simulink model "pid_pith"  (Simulink 5.0)
settings: Solver=ode5  StartTime=0.0  StopTime=75  FixedStep=.01  RelTol=1e-3
values from neighbouring files (symbols this model uses):
  control_p = [-1 -0.975 -0.95 -0.925 -0.9 -0.875 -0.85 -0.825 -0.8 -0.775 -0.75 -0.725 ... (81 elements, 1x81)]    [tras_char.mat]
  force_p = [-0.71417078206 -0.698541481137 -0.676359428972 -0.657306593399 -0.636149510201 -0.615949677515 -0.602138570677 -0.585879142379 -0.565408182885 -0.543655801355 -0.527755120628 -0.502405059235 ... (81 elements, 1x81)]    [tras_char.mat]
  rpm_p = [-3678.29210985 -3557.9090356 -3500.75969748 -3468.48920637 -3408.40308809 -3364.59631401 -3305.24812764 -3268.16062475 -3204.9654373 -3137.29807834 -3101.82489983 -3044.64042209 ... (81 elements, 1x81)]    [tras_char.mat]
undefined symbols (not defined in the file or in its folder): a, b, c
settings Model: LastModifiedBy=Administrator

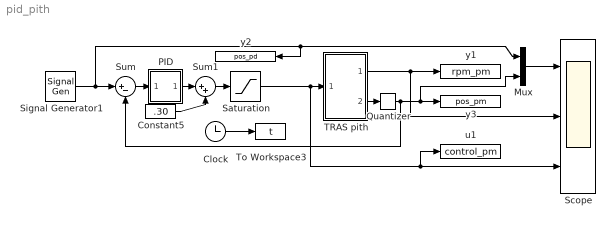
== system pid_pith ==
  Clock : Clock
  Constant5 : Constant  Value=.30
  Mux : Mux  Inputs=2
  "PID " : Subsystem  AncestorBlock=|  mask(PID(2) Controller){P=a, I=b, D=c, N=100, S=1.43}
      | simulink_extras/Additional
      | Linear/PID Controller
      | (with Approximate
      | Derivative)
      mask prompts: P "Proportional:"; I "Integral:"; D "Derivative:"; N "Derivative divisor(N):"; S "Integral sat (0-1)"
      mask help:
      | Enter Proportional(P), Integral(I), and Derivative(D) and divisor (N) terms.
      | P+I/s+Ds/(1/Ns+1)
      mask Help: This block implements a PID controller where parameters are entered for the Proportional, Integral and Derivative and divisor terms. Unmask this block to see how it works. The derivative term is implemented using an s/(s/N +1)  transfer function block. Making N large can create a "stiff" system.
      mask Display: disp('PID')
  Quantizer : Quantizer  QuantizationInterval=(2*pi)/4096
  Saturation : Saturate  UpperLimit=1  LowerLimit=.2
  Scope : Scope  NumInputPorts=3
      settings: YMin=-1.5~0~0  YMax=1~3000~1  MaxDataPoints=50000
  Signal Generator1 : SignalGenerator  WaveForm=square  Amplitude=.10  Frequency=.02
  Sum : Sum  Inputs=|+-  SaturateOnIntegerOverflow=on
  Sum1 : Sum  Inputs=|++  SaturateOnIntegerOverflow=on  InputSameDT=on
  TRAS pith : Subsystem
  To Workspace3 : ToWorkspace  VariableName=t  SampleTime=-1  SaveFormat=Array
  u1 : ToWorkspace  VariableName=control_pm  SampleTime=-1  SaveFormat=Array
  y1 : ToWorkspace  VariableName=rpm_pm  SampleTime=-1  SaveFormat=Array
  y2 : ToWorkspace  VariableName=pos_pd  SampleTime=-1  SaveFormat=Array
  y3 : ToWorkspace  VariableName=pos_pm  SampleTime=-1  SaveFormat=Array
  wires:
  TRAS pith/1(rpm_p) -> y1/1, Scope/2
  TRAS pith/2(pos_pm) -> Quantizer/1
  Clock/1 -> To Workspace3/1
  Signal Generator1/1 -> Sum/1, Mux/1, y2/1
  Sum/1 -> "PID "/1(In_1)
  Mux/1 -> Scope/1
  Saturation/1 -> TRAS pith/1(ctrl_p), Scope/3, u1/1
  "PID "/1(Out_1) -> Sum1/1
  Sum1/1 -> Saturation/1
  Constant5/1 -> Sum1/2
  Quantizer/1 -> y3/1, Mux/2, Sum/2

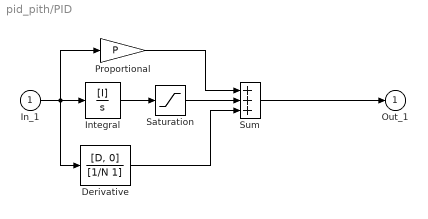
== system pid_pith/PID  ==
  In_1 : Inport
  Derivative : TransferFcn  Numerator=[D, 0]  Denominator=[1/N 1]
  Integral : TransferFcn  Numerator=[I]  Denominator=[1 0]
  Proportional : Gain  Gain=P  SaturateOnIntegerOverflow=on
  Saturation : Saturate  UpperLimit=S  LowerLimit=-S
  Sum : Sum  Inputs=+++  SaturateOnIntegerOverflow=on  InputSameDT=on
  Out_1 : Outport  InitialOutput=0
  wires:
  Sum/1 -> Out_1/1
  In_1/1 -> Derivative/1, Integral/1, Proportional/1
  Derivative/1 -> Sum/3
  Integral/1 -> Saturation/1
  Proportional/1 -> Sum/1
  Saturation/1 -> Sum/2

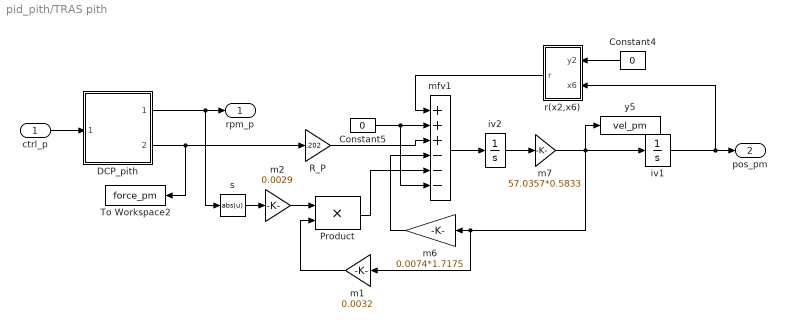
== system pid_pith/TRAS pith ==
  ctrl_p : Inport
  Constant4 : Constant  Orientation=left  Value=0
  Constant5 : Constant  Value=0
  DCP_pith : Subsystem
  Product : Product  SaturateOnIntegerOverflow=on
  R_P : Gain  Gain=.202
  To Workspace2 : ToWorkspace  VariableName=force_pm  SampleTime=-1  SaveFormat=Array
  iv1 : Integrator  InitialCondition=-.5319*0  UpperSaturationLimit=pi  LowerSaturationLimit=-pi
  iv2 : Integrator  InitialCondition=-.1  LimitOutput=on  UpperSaturationLimit=pi  LowerSaturationLimit=-pi
  m1 : Gain  Orientation=left  Gain=0.0032  SaturateOnIntegerOverflow=on
  m2 : Gain  Gain=0.0029  SaturateOnIntegerOverflow=on
  m6 : Gain  Orientation=left  Gain=0.0074*1.7175
  m7 : Gain  Gain=57.0357*0.5833  SaturateOnIntegerOverflow=on
  mfv1 : Sum  Inputs=+++---  SaturateOnIntegerOverflow=on  InputSameDT=on
  r(x2,x6) : Subsystem  Orientation=left
  s : Fcn  Expr=abs(u)
  y5 : ToWorkspace  VariableName=vel_pm  SampleTime=-1  SaveFormat=Array
  rpm_p : Outport
  pos_pm : Outport  Port=2
  wires:
  ctrl_p/1 -> DCP_pith/1(CTR_P)
  mfv1/1 -> iv2/1
  m2/1 -> Product/1
  m1/1 -> Product/2
  iv1/1 -> pos_pm/1, r(x2,x6)/2(x6)
  Constant5/1 -> mfv1/6, mfv1/2
  Constant4/1 -> r(x2,x6)/1(y2)
  R_P/1 -> mfv1/3
  r(x2,x6)/1(r) -> mfv1/1
  Product/1 -> mfv1/5
  s/1 -> m2/1
  DCP_pith/1(RPM_P) -> rpm_p/1, s/1
  m7/1 -> iv1/1, m1/1, m6/1, y5/1
  iv2/1 -> m7/1
  m6/1 -> mfv1/4
  DCP_pith/2(FORCE_P) -> R_P/1, To Workspace2/1

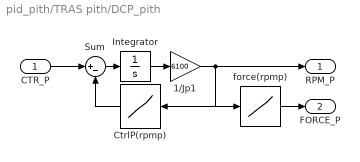
== system pid_pith/TRAS pith/DCP_pith ==
  CTR_P : Inport
  1/Jp1 : Gain  Gain=6100  ShowAdditionalParam=on
  CtrlP(rpmp) : Lookup  Orientation=left  InputValues=rpm_p  OutputValues=control_p  SaturateOnIntegerOverflow=on
  Integrator : Integrator
  Sum : Sum  Inputs=|+-  SaturateOnIntegerOverflow=on  InputSameDT=on
  force(rpmp) : Lookup  InputValues=rpm_p  OutputValues=force_p  SaturateOnIntegerOverflow=on
  RPM_P : Outport
  FORCE_P : Outport  Port=2
  wires:
  force(rpmp)/1 -> FORCE_P/1
  CTR_P/1 -> Sum/1
  1/Jp1/1 -> RPM_P/1, force(rpmp)/1, CtrlP(rpmp)/1
  CtrlP(rpmp)/1 -> Sum/2
  Integrator/1 -> 1/Jp1/1
  Sum/1 -> Integrator/1

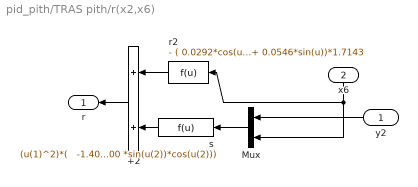
== system pid_pith/TRAS pith/r(x2,x6) ==
  y2 : Inport  Orientation=left
  x6 : Inport  Orientation=down  Port=2
  +2 : Sum  Orientation=left  SaturateOnIntegerOverflow=on  InputSameDT=on
  Mux : Mux  Orientation=left  Inputs=2
  r2 : Fcn  Orientation=left  Expr=- ( 0.0292*cos(u)+ 0.0546*sin(u))*1.7143
  s : Fcn  Orientation=left  Expr="(u(1)^2)*(   -1.40920355960000 *sin(u(2))*cos(u(2)))"
  r : Outport  Orientation=left
  wires:
  +2/1 -> r/1
  y2/1 -> Mux/1
  x6/1 -> r2/1, Mux/2
  s/1 -> +2/2
  r2/1 -> +2/1
  Mux/1 -> s/1
